simulink model "ONE"  (R2020a)
settings: Solver=VariableStepAuto  StartTime=0.0  StopTime=40  RelTol=1e-3
libraries: powerlib x6, simulink x3
settings Model: Creator=lai  LastModifiedBy=lai

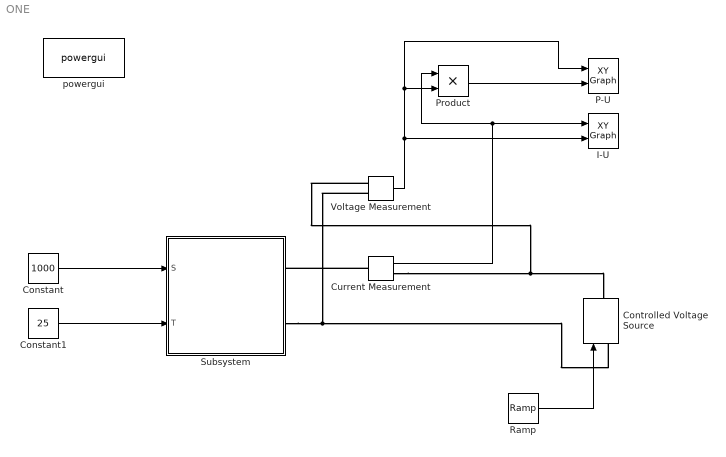
== system ONE ==
  Constant : Constant  Value=1000
  Constant1 : Constant  Value=25
  Controlled Voltage Source : powerlib/Electrical Sources/Controlled Voltage Source  Initialize=on  Source_Type=AC  Amplitude=0  Phase=0  Frequency=0  Measurements=None
  Current Measurement : powerlib/Measurements/Current Measurement  PhasorSimulation=off  OutputType=Complex  PSBequivalent=0
  I-U : simulink/Sinks/XY Graph  xmin=0  xmax=10  ymin=0  ymax=40  st=-1
  P-U : simulink/Sinks/XY Graph  xmin=0  xmax=40  ymin=0  ymax=400  st=-1
  Product : Product
  Ramp : simulink/Sources/Ramp  slope=40  start=0  InitialOutput=0
  Subsystem : Subsystem  mask{Uoc=36.3, Um=29, Isc=7.84, Im=7.35}
  Voltage Measurement : powerlib/Measurements/Voltage Measurement  PhasorSimulation=off  OutputType=Complex  PSBequivalent=0
  powergui : powerlib/powergui  Priority=1  SimulationMode=Discrete  SampleTime=0.005  frequency=60  Iterations=50  frequencyindice=0  Pbase=100e6  ErrMax=1e-4  UnitsV=kV  UnitsW=MW  buscounter=0  FunctionMessages=off  echomessages=off  EnableUseOfTLC=off  CurrentSourceSwitches=off  DisableSnubberDevices=off  DisableRonSwitches=off  DisableVfSwitches=off  DisplayEquations=off  AutomaticDiscreteSolvers=off  SolverType=Tustin/Backward Euler (TBE)  Interpol=off  ExternalGateDelay=off  methode=off  Ts=100  x0status=blocks  SPID=on  SwTol=0  HookPort=off  NonlinearTolerance=1e-4  nMaxIteration=100  ContinueOnMaxIteration=off  RestoreLinks=warning  ResistiveCurrentMeasurement=off  Frange=[0:2:500]  Ylog=off  Xlog=on  ShowGrid=off  save=off  variable=ZData  structure=0  ZoomFFT=off  StartTime=0.0  cycles=1  DisplayStyle=1  fundamental=60  FreqAxis=off  MaxFrequency=1000  frequencyindicesteady=1  RmsSteady=1  display=off
  wires:
  Constant/1 -> Subsystem/1(S)
  Constant1/1 -> Subsystem/2(T)
  Product/1 -> P-U/2
  Voltage Measurement/1 -> Product/2, P-U/1, I-U/2
  Current Measurement/1 -> Product/1, I-U/1
  Ramp/1 -> Controlled Voltage Source/1
  connections:
  Current Measurement/LConn1 -- Subsystem/RConn1
  Current Measurement/RConn1 -- Voltage Measurement/LConn1 -- Controlled Voltage Source/RConn1
  Subsystem/RConn2 -- Controlled Voltage Source/LConn1 -- Voltage Measurement/LConn2

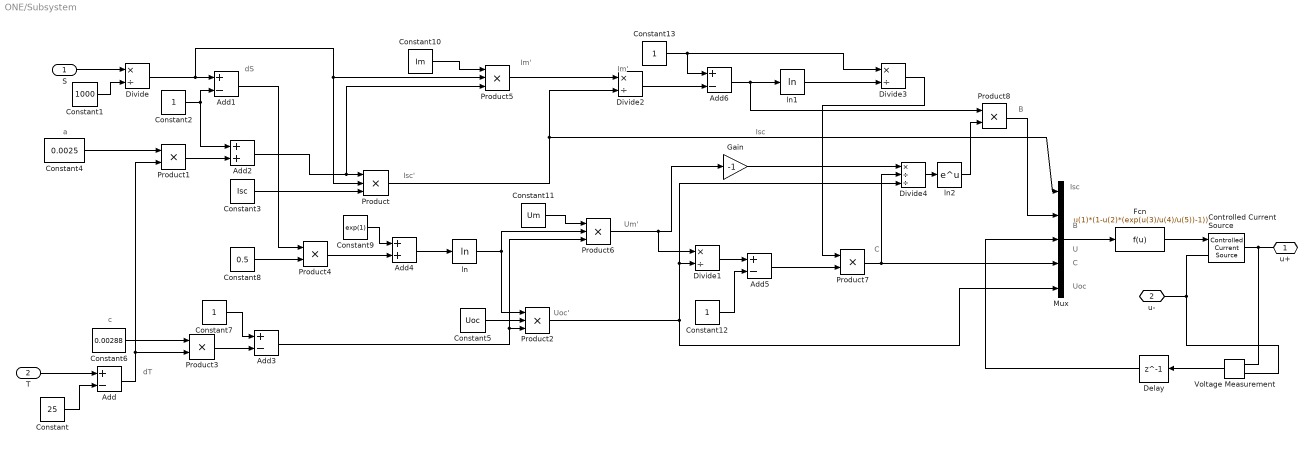
== system ONE/Subsystem ==
  note: c
  note: a
  note: Isc'
  note: dS
  note: dT
  note: Isc
  note: B
  note: U
  note: C
  note: Uoc
  note: Uoc'
  note: Im'
  note: Um'
  note: C
  note: B
  note: Isc
  note: Im'
  S : Inport
  T : Inport  Port=2
  Add{,1,3,5..6} (5 alike) : Sum  Inputs=+-
  Add2 : Sum
  Add4 : Sum
  Constant : Constant  Value=25
  Constant1 : Constant  Value=1000
  Constant10 : Constant  Value=Im
  Constant11 : Constant  Value=Um
  Constant{2,7,12..13} (4 alike) : Constant
  Constant3 : Constant  Value=Isc
  Constant4 : Constant  Value=0.0025
  Constant5 : Constant  Value=Uoc
  Constant6 : Constant  Value=0.00288
  Constant8 : Constant  Value=0.5
  Constant9 : Constant  Value=exp(1)
  Controlled Current Source : powerlib/Electrical Sources/Controlled Current Source  Initialize=on  Source_Type=DC  Amplitude=0  Phase=0  Frequency=0  Measurements=None
  Delay : Delay  DelayLength=1
  Divide{,1..3} (4 alike) : Product  Inputs=*/
  Divide4 : Product  Inputs=*//
  Fcn : Fcn  Expr=u(1)*(1-u(2)*(exp(u(3)/u(4)/u(5))-1))
  Gain : Gain  Gain=-1
  Mux : Mux  Inputs=5
  Product{,2,5..6} (4 alike) : Product  Inputs=3
  Product{1,3..4,7..8} (5 alike) : Product
  Voltage Measurement : powerlib/Measurements/Voltage Measurement  PhasorSimulation=off  OutputType=Complex  PSBequivalent=0
  ln : Math  Operator=log  SaturateOnIntegerOverflow=on
  ln1 : Math  Operator=log  SaturateOnIntegerOverflow=on
  ln2 : Math  SaturateOnIntegerOverflow=on
  " u+" : PMIOPort  Side=Right
  " u-" : PMIOPort  Port=2  Side=Right
  wires:
  Fcn/1 -> Controlled Current Source/1
  Mux/1 -> Fcn/1
  T/1 -> Add/1
  Constant/1 -> Add/2
  S/1 -> Divide/1
  Constant1/1 -> Divide/2
  Divide/1 -> Product/2, Product5/2, Add1/1
  Constant2/1 -> Add2/1, Add1/2
  Product1/1 -> Add2/2
  Add/1 -> Product3/2, Product1/2
  Constant4/1 -> Product1/1
  Constant3/1 -> Product/3
  Add2/1 -> Product5/3, Product/1
  Constant6/1 -> Product3/1
  Product3/1 -> Add3/2
  Constant7/1 -> Add3/1
  Add3/1 -> Product6/3, Product2/3
  Constant5/1 -> Product2/2
  Constant8/1 -> Product4/2
  Product4/1 -> Add4/2
  Add4/1 -> ln/1
  ln/1 -> Product6/2, Product2/1
  Constant9/1 -> Add4/1
  Constant10/1 -> Product5/1
  Add1/1 -> Product4/1
  Constant11/1 -> Product6/1
  Product6/1 -> Gain/1, Divide1/1
  Product2/1 -> Divide4/3, Divide1/2, Mux/5
  Divide1/1 -> Add5/1
  Constant12/1 -> Add5/2
  Add5/1 -> Product7/2
  Product/1 -> Divide2/2, Mux/1
  Product5/1 -> Divide2/1
  Divide2/1 -> Add6/2
  Constant13/1 -> Divide3/1, Add6/1
  Add6/1 -> ln1/1, Product8/1
  ln1/1 -> Divide3/2
  Divide3/1 -> Product7/1
  Product7/1 -> Divide4/2, Mux/4
  Gain/1 -> Divide4/1
  Divide4/1 -> ln2/1
  ln2/1 -> Product8/2
  Product8/1 -> Mux/2
  Delay/1 -> Mux/3
  Voltage Measurement/1 -> Delay/1
  connections:
  " u-"/RConn1 -- Controlled Current Source/LConn1 -- Voltage Measurement/LConn2
  Controlled Current Source/RConn1 -- Voltage Measurement/LConn1 -- " u+"/RConn1
